simulink model "Peacemaker"  (R2020a)
settings: Solver=FixedStepAuto  StartTime=0.0  StopTime=10.0  FixedStep=1e-3  RelTol=1e-3  EnableMultiTasking=on
undefined symbols (not defined in the file): D0, D1, D10, D11, D12, D13, D2, D3, D4, D5, D6, D7, D8, D9, PTA0, PTA1, PTA2, PTB23, PTB9, PTC16, PTC17, PTC2, PTC3, PTC4, PTD0, PTD1, PTD2, PTD3
libraries: frdmk64flib x14
settings Model: ExtModeTrigDuration=5  Creator=sxj  LastModifiedBy=sxj
settings OptimizationCC: EnhancedBackFolding=on  PassReuseOutputArgsAs=Individual arguments  ZeroExternalMemoryAtStartup=off  ZeroInternalMemoryAtStartup=off  MaxStackSize=64  OptimizeBlockOrder=speed  DifferentSizesBufferReuse=on  OptimizationCustomize=off  EfficientTunableParamExpr=on
settings DebuggingCC: ParameterTunabilityLossMsg=error
settings HardwareCC: ProdBitPerPointer=32  ProdBitPerSizeT=32  ProdBitPerPtrDiffT=32  ProdLargestAtomicInteger=Long  ProdLargestAtomicFloat=Double  ProdWordSize=32  ProdHWDeviceType=ARM Compatible->ARM Cortex
settings SFSimCC: MATLABDynamicMemAlloc=off
settings RTWCC: SystemTargetFile=ert.tlc  HardwareBoard=NXP FRDM-K64F  TemplateMakefile=ert_default_tmf  Toolchain=GNU Tools for ARM Embedded Processors
settings CodeAppCC: ForceParamTrailComments=on  IgnoreCustomStorageClasses=off  OperatorAnnotations=on  SimulinkDataObjDesc=on  SFDataObjDesc=on  InsertBlockDesc=on

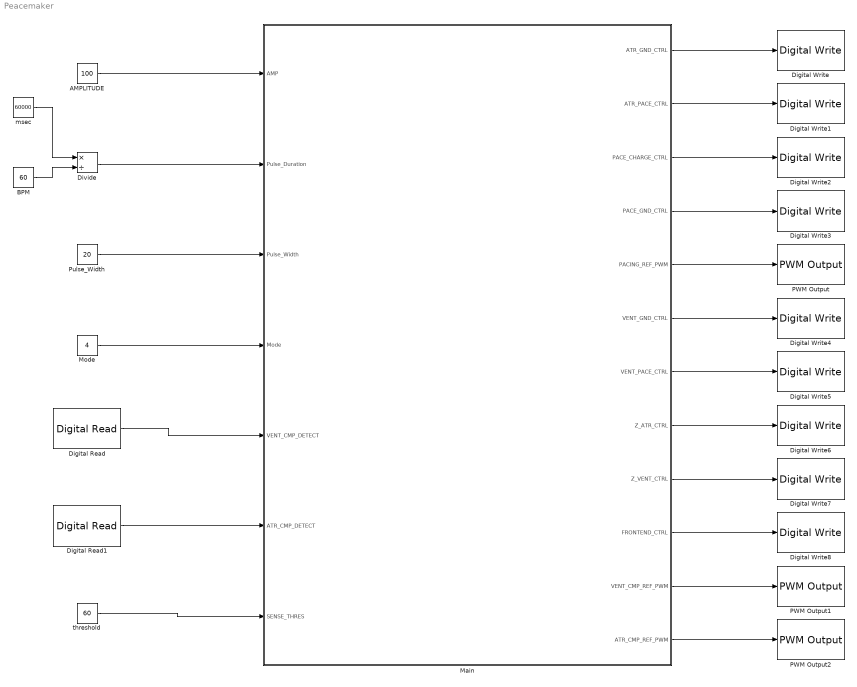
== system Peacemaker ==
  AMPLITUDE : Constant  Value=100
  BPM : Constant  Value=60
  Digital Read : frdmk64flib/Digital Read  Whichpin=PTC17 (D1)  SampleTime=-1
  Digital Read1 : frdmk64flib/Digital Read  Whichpin=PTC16 (D0)  SampleTime=-1
  Digital Write : frdmk64flib/Digital Write  Whichpin=PTD2 (D11)
  Digital Write1 : frdmk64flib/Digital Write  Whichpin=PTA0 (D8)
  Digital Write2 : frdmk64flib/Digital Write  Whichpin=PTB9 (D2)
  Digital Write3 : frdmk64flib/Digital Write  Whichpin=PTD0 (D10)
  Digital Write4 : frdmk64flib/Digital Write  Whichpin=PTD3 (D12)
  Digital Write5 : frdmk64flib/Digital Write  Whichpin=PTC4 (D9)
  Digital Write6 : frdmk64flib/Digital Write  Whichpin=PTB23 (D4)
  Digital Write7 : frdmk64flib/Digital Write  Whichpin=PTC3 (D7)
  Digital Write8 : frdmk64flib/Digital Write  Whichpin=PTD1 (D13)
  Divide : Product  Inputs=*/
  Main : Stateflow chart  TreatAsAtomicUnit=on
  Mode : Constant  Value=4
  PWM Output : frdmk64flib/PWM Output  Whichpin=PTA2 (D5)  InitialFrequency=2000  InitialDutyCycle=0
  PWM Output1 : frdmk64flib/PWM Output  Whichpin=PTA1 (D3)  InitialFrequency=2000  InitialDutyCycle=0
  PWM Output2 : frdmk64flib/PWM Output  Whichpin=PTC2 (D6)  InitialFrequency=2000  InitialDutyCycle=0
  Pulse_Width : Constant  Value=20
  msec : Constant  Value=60000
  threshold : Constant  Value=60
  wires:
  AMPLITUDE/1 -> Main/1(AMP)
  msec/1 -> Divide/1
  BPM/1 -> Divide/2
  Divide/1 -> Main/2(Pulse_Duration)
  Pulse_Width/1 -> Main/3(Pulse_Width)
  Mode/1 -> Main/4(Mode)
  Main/1(ATR_GND_CTRL) -> Digital Write/1
  Main/2(ATR_PACE_CTRL) -> Digital Write1/1
  Main/3(PACE_CHARGE_CTRL) -> Digital Write2/1
  Main/4(PACE_GND_CTRL) -> Digital Write3/1
  Main/5(PACING_REF_PWM) -> PWM Output/1
  Main/6(VENT_GND_CTRL) -> Digital Write4/1
  Main/7(VENT_PACE_CTRL) -> Digital Write5/1
  Main/8(Z_ATR_CTRL) -> Digital Write6/1
  Main/9(Z_VENT_CTRL) -> Digital Write7/1
  Digital Read1/1 -> Main/6(ATR_CMP_DETECT)
  Digital Read/1 -> Main/5(VENT_CMP_DETECT)
  Main/10(FRONTEND_CTRL) -> Digital Write8/1
  threshold/1 -> Main/7(SENSE_THRES)
  Main/11(VENT_CMP_REF_PWM) -> PWM Output1/1
  Main/12(ATR_CMP_REF_PWM) -> PWM Output2/1

== stateflow chart Peacemaker/Main ==
  state AOO
    state AOO_CHARGE
      entry:
      PACING_REF_PWM = AMP;
      PACE_CHARGE_CTRL = 1;
      ATR_PACE_CTRL = 0;
      ATR_GND_CTRL = 1;
      PACE_GND_CTRL = 0;
      Z_ATR_CTRL = 0;
    state AOO_PACE
      entry:
      PACING_REF_PWM = AMP;
      PACE_CHARGE_CTRL = 0;
      ATR_PACE_CTRL = 1;
      ATR_GND_CTRL = 0;
      PACE_GND_CTRL = 1;
      Z_ATR_CTRL = 0;
    (default) -> AOO_CHARGE
    AOO_CHARGE -> AOO_PACE : after(Pulse_Duration-Pulse_Width,msec)
    AOO_PACE -> AOO_CHARGE : after(Pulse_Width,msec)
  state VVI
    state VVI_CHARGE
      entry:
      PACING_REF_PWM = AMP;
      PACE_CHARGE_CTRL = 1;
      VENT_PACE_CTRL = 0;
      VENT_GND_CTRL = 1;
      PACE_GND_CTRL = 0;
      Z_VENT_CTRL = 0;
      FRONTEND_CTRL = 1;
      VENT_CMP_REF_PWM = SENSE_THRES;
    state VVI_PACE
      entry:
      PACING_REF_PWM = AMP;
      PACE_CHARGE_CTRL = 0;
      VENT_PACE_CTRL = 1;
      VENT_GND_CTRL = 0;
      PACE_GND_CTRL = 1;
      Z_VENT_CTRL = 0;
      FRONTEND_CTRL = 1;
      VENT_CMP_REF_PWM = SENSE_THRES;
    (junction 55) -> VVI_CHARGE [order 2] : [VENT_CMP_DETECT == 1]
    (default) -> VVI_CHARGE
    VVI_CHARGE -> (junction 55)
    (junction 55) -> VVI_PACE [order 1] : after(Pulse_Duration-Pulse_Width,msec)[VENT_CMP_DETECT == 0]
    VVI_PACE -> VVI_CHARGE : after(Pulse_Width,msec)
  state AAI
    state AAI_CHARGE
      entry:
      PACING_REF_PWM = AMP;
      PACE_CHARGE_CTRL = 1;
      ATR_PACE_CTRL = 0;
      ATR_GND_CTRL = 1;
      PACE_GND_CTRL = 0;
      Z_ATR_CTRL = 0;
      FRONTEND_CTRL = 1;
      ATR_CMP_REF_PWM = SENSE_THRES;
    state AAI_PACE
      entry:
      PACING_REF_PWM = AMP;
      PACE_CHARGE_CTRL = 0;
      ATR_PACE_CTRL = 1;
      ATR_GND_CTRL = 0;
      PACE_GND_CTRL = 1;
      Z_ATR_CTRL = 0;
      FRONTEND_CTRL = 1;
      ATR_CMP_REF_PWM = SENSE_THRES;
    (junction 49) -> AAI_CHARGE [order 2] : [ATR_CMP_DETECT == 1]
    (default) -> AAI_CHARGE
    AAI_CHARGE -> (junction 49)
    (junction 49) -> AAI_PACE [order 1] : after(Pulse_Duration-Pulse_Width,msec)[ATR_CMP_DETECT == 0]
    AAI_PACE -> AAI_CHARGE : after(Pulse_Width,msec)
  state IDLE_STATE
  state VOO
    state VOO_CHARGE
      entry:
      PACING_REF_PWM = AMP;
      PACE_CHARGE_CTRL = 1;
      VENT_PACE_CTRL = 0;
      VENT_GND_CTRL = 1;
      PACE_GND_CTRL = 0;
      Z_VENT_CTRL = 0;
    state VOO_PACE
      entry:
      PACING_REF_PWM = AMP;
      PACE_CHARGE_CTRL = 0;
      VENT_PACE_CTRL = 1;
      VENT_GND_CTRL = 0;
      PACE_GND_CTRL = 1;
      Z_VENT_CTRL = 0;
    (default) -> VOO_CHARGE
    VOO_CHARGE -> VOO_PACE : after(Pulse_Duration-Pulse_Width,msec)
    VOO_PACE -> VOO_CHARGE : after(Pulse_Width,msec)
  IDLE_STATE -> AOO [order 1] : [Mode == 0]
  AOO -> IDLE_STATE : [Mode ~= 0]
  (default) -> IDLE_STATE
  IDLE_STATE -> VVI [order 4] : [Mode == 4]
  IDLE_STATE -> AAI [order 3] : [Mode == 3]
  AAI -> IDLE_STATE : [Mode ~= 3]
  VVI -> IDLE_STATE : [Mode ~= 4]
  IDLE_STATE -> VOO [order 2] : [Mode == 1]
  VOO -> IDLE_STATE : [Mode ~= 1]
  data: AMP input; ATR_GND_CTRL output; ATR_PACE_CTRL output; PACE_CHARGE_CTRL output; PACE_GND_CTRL output; PACING_REF_PWM output; VENT_GND_CTRL output; VENT_PACE_CTRL output; Z_ATR_CTRL output; Z_VENT_CTRL output; Pulse_Duration input; Pulse_Width input; Mode input; FRONTEND_CTRL output; VENT_CMP_DETECT input; ATR_CMP_DETECT input; SENSE_THRES input; VENT_CMP_REF_PWM output; ATR_CMP_REF_PWM output
